simulink model "buttonblink_task"  (Simulink 3.00)
libraries: genlib x2, mathlib x2, logiclib x1

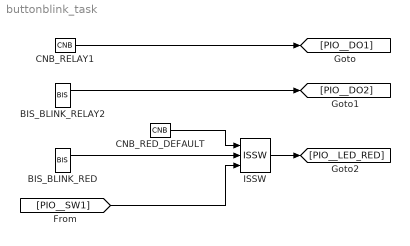
== system buttonblink_task ==
  BIS_BLINK_RED : genlib/BIS  Y0=off  t1=0.2  t2=0.4  t3=0  t4=0  t5=0  t6=0  t7=2.0  t8=0  RPT=on  bEdit=off
  BIS_BLINK_RELAY2 : genlib/BIS  Y0=off  t1=1  t2=2  t3=0  t4=4  t5=5  t6=6  t7=7  t8=8  RPT=on  bEdit=off
  CNB_RED_DEFAULT : mathlib/CNB  YCN=off
  CNB_RELAY1 : mathlib/CNB  YCN=on
  ISSW : logiclib/ISSW
  wires:
  BIS_BLINK_RELAY2/1 -> [PIO__DO2]
  BIS_BLINK_RED/1 -> ISSW/2
  CNB_RELAY1/1 -> [PIO__DO1]
  CNB_RED_DEFAULT/1 -> ISSW/1
  [PIO__SW1] -> ISSW/3
  ISSW/1 -> [PIO__LED_RED]
